simulink model "resultados_controle_FALA_tuned_PID"  (Simulink 8.7)
settings: Solver=ode45  StartTime=0.0  StopTime=260  FixedStep=0.01  MaxStep=0.1  RelTol=1e-3
InitFcn:
  | % load parameters of the default quadrotor
  | disp('Quadrotor parameters loaded by InitFcn')
  | load =250;
  | mdl_quadrotor
  | 
  | % --- Outer loop gains --------
  | %Versao 1
  | %P_X = 3.25; I_X = 0.45; D_X = 2;
  | %P_Y = 2.75; I_Y = 0.35; D_Y = 4.75;
  | %P_Z = 45;    I_Z = 3.5;   D_Z = 25;
  | 
  | %FALA TUNNED WITH LOAD
  | P_X = 9.2;      I_X = 0.16;     D_X  =  3.45;
  | P_Y = 8.9;      I_Y = 0.04;      D_Y  = 3.5;
  | P_Z = 53;       I_Z = 5.2;        D_Z = 26.7;
  | % --------------------------
undefined symbols (not defined in the file or in its folder): quad, sigbuilder_block
libraries: simulink_extras x5, dspsigops x4
settings Model: Creator=corkep  LastModifiedBy=kleber
settings DataIOCC: SignalLoggingSaveFormat=ModelDataLogs
settings OptimizationCC: ExpressionDepthLimit=2147483647
settings DebuggingCC: SolverPrmCheckMsg=warning  FcnCallInpInsideContextMsg=UseLocalSettings  StateNameClashWarn=warning
settings GRTTargetCC: CombineOutputUpdateFcns=off  GRTInterface=on
settings ConfigComp: CovSFcnEnable=off

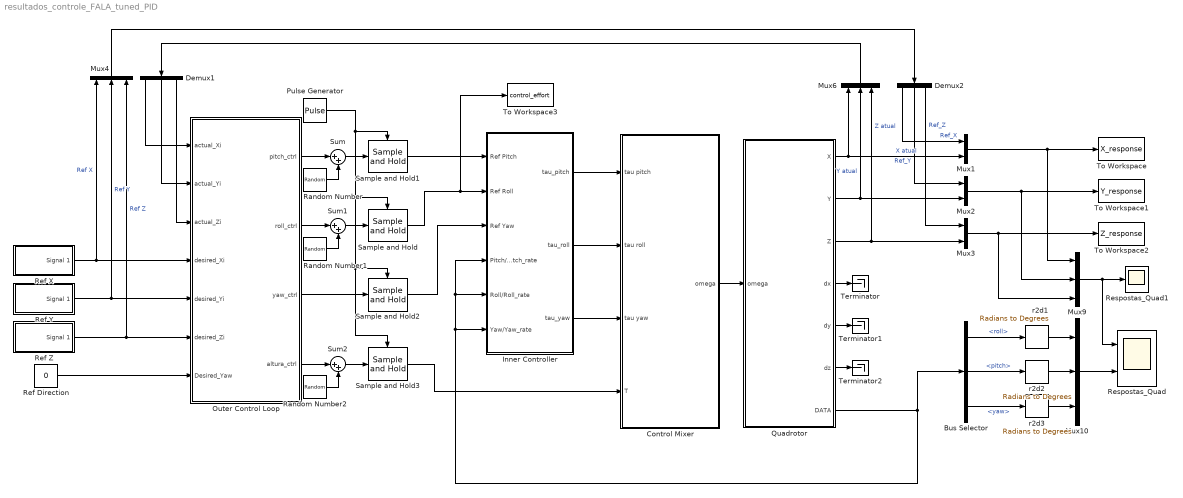
== system resultados_controle_FALA_tuned_PID ==
  Bus Selector : BusSelector  OutputSignals=roll,pitch,yaw
  Control Mixer : Subsystem  AncestorBlock=roblocks/Dynamics/Control Mixer 4
      mask help: Quadrotor control mixer
      mask Help:
      | Determine rotor speeds based on desired torques and thrust.
      | 
      | <b>Inputs::</b>
      | 
      | tau pitch (1x1)  desired pitching torque [Nm]
      | tau roll (1x1)   desired rolling torque [Nm]
      | tau yaw (1x1)    desired yawing torque [Nm]
      | T (1x1)          desired thrust [N]
      | 
      | <b>Outputs::</b>
      | 
      | w1 (1x1) angular velocity of rotor 1 [rad]
      | w2 (1x1) angular velocity of rotor 2 [rad]
      | w3 (1x1) angular velocity of rotor 3 [rad]
      | w4 (1x1) angular velocity of rotor 4 [rad]
      | 
      | <b>Notes::</b>
      | 
      | - Assumes the rotor labelling convention of RVC Fig 4.16.
      | - The quadrotor is underactuated and has only 4 inputs.
  Demux1 : Demux  Outputs=3
  Demux2 : Demux  Outputs=3
  Inner Controller : Subsystem
  Mux1 : Mux  Inputs=2
  Mux10 : Mux  Inputs=3
  Mux2 : Mux  Inputs=2
  Mux3 : Mux  Inputs=2
  Mux4 : Mux  Inputs=3
  Mux6 : Mux  RequirementInfo="{}  %GIDa_c1e701bd_0944_43f7_91ee_3360df493ed1"  Inputs=3
  Mux9 : Mux  Inputs=3
  Outer Control Loop : Subsystem
  Pulse Generator : DiscretePulseGenerator  PulseType=Time based  Period=0.1  PulseWidth=10
  Quadrotor : Subsystem  AncestorBlock=roblocks/Dynamics/Quadrotor  mask{quad=quad}
      mask prompts: quad "Quadrotor params"
      mask help: Quadrotor dynamics
      mask Help:
      | Integrate spatial velocity to update pose represented as a homogeneous
      | transformation.
      | 
      | <b>Parameters::</b>
      | 
      | q (struct)  A structure containing quadrotor dynamics
      | 
      | The elements of q are:
      | 
      |  J         Flyer rotational inertia matrix (3x3)
      |  h         Height of rotors above CoG (1x1)
      |  d         Length of flyer arms (1x1)
      |  nb        Number of blades per rotor (1x1)
      |  r         Rotor radius (1x1)
      |  c         Blade chord (1x1)
      |  e         Flapping hinge offset (1x1)
      |  Mb        Rotor blade mass (1x1)
      |  Mc        Estimated hub clamp mass (1x1)
      |  ec        Blade root clamp displacement (1x1)
      |  Ib        Rotor blade rotational inertia (1x1)
      |  Ic        Estimated root clamp inertia (1x1)
      |  mb        Static blade moment (1x1)
      |  Ir        Total rotor inertia (1x1)
      |  Ct        Non-dim. thrust coefficient (1x1)
      |  Cq        Non-dim. torque coefficient (1x1)
      |  sigma     Rotor solidity ratio (1x1)
      |  thetat    Blade tip angle (1x1)
      |  theta0    Blade root angle (1x1)
      |  theta1    Blade twist angle (1x1)
      |  theta75   3/4 blade angle (1x1)
      |  thetai    Blade ideal root approximation (1x1)
      |  a         Lift slope gradient (1x1)
      |  A         Rotor disc area (1x1)
      |  gamma     Lock number (1x1)
      | 
      | 
      | <b>Inputs::</b>
      | 
      | w1 (1x1) angular velocity of rotor 1 [rad]
      | w2 (1x1) angular velocity of rotor 2 [rad]
      | w3 (1x1) angular velocity of rotor 3 [rad]
      | w4 (1x1) angular velocity of rotor 4 [rad]
      | 
      | <b>Outputs::</b>
      | 
      | X (1x12) state vector (x, y, z, thr, thp, thy, xd, yd, zd, thrd, thpd, thyd)
      | 
      | (x,y,z) is the position in the world frame [m]
      | (thr, thp, thy) the roll/pitch/yaw orientation in the world frame [rad]
      | (xd,yd,zd) is the velocity in the body frame [m]
      | (thrd,thpd,thyd) is the roll/pitch/yaw rates in the body frame [rad/s]
      | 
      | <b>Notes::</b>
      | 
      | - See also mdl_quadrotor which defines parameters for the ANU X4 flyer.
  Random Number : RandomNumber  Variance=0.0001  SampleTime=0.01
  Random Number1 : RandomNumber  Variance=0.0001  SampleTime=0.01
  Random Number2 : RandomNumber  Variance=0.25  SampleTime=0.01
  Ref Direction : Constant  Value=0  SampleTime=0
  Ref X : Subsystem  Tag=STV Subsys  LoadFcn=sigbuilder_block('load');  StartFcn=sigbuilder_block('start');  StopFcn=sigbuilder_block('stop');  ClipboardFcn=sigbuilder_block('clipboard');  mask(Sigbuilder block){}
      mask help: Sigbuilder GUI
      mask init:
      | if ~strcmp(get_param(bdroot(gcbh),'SimulationStatus'),'stopped') tuvar = sigbuilder_block('maskInit'); end
      settings: CopyFcn=sigbuilder_block('copy');  DeleteFcn=sigbuilder_block('delete');  ModelCloseFcn=sigbuilder_block('modelClose');  PreSaveFcn=sigbuilder_block('preSave');  PauseFcn=sigbuilder_block('pause')  ContinueFcn=sigbuilder_block('continue')  NameChangeFcn=sigbuilder_block('namechange');  OpenFcn=sigbuilder_block('open',[156 64.5 984.75 417 ]);  CloseFcn=sigbuilder_block('close');
      mask Display: plot(0,0,100,100,[10,10,40,40,10],[80,20,20,80,80],[40,10],[50,50], [40,27,10],[65,72,56],[40,25,25,10],[28,28,43,43]);
  Ref Y : Subsystem  Tag=STV Subsys  LoadFcn=sigbuilder_block('load');  StartFcn=sigbuilder_block('start');  StopFcn=sigbuilder_block('stop');  ClipboardFcn=sigbuilder_block('clipboard');  mask(Sigbuilder block){}
      mask help: Sigbuilder GUI
      mask init:
      | if ~strcmp(get_param(bdroot(gcbh),'SimulationStatus'),'stopped') tuvar = sigbuilder_block('maskInit'); end
      settings: CopyFcn=sigbuilder_block('copy');  DeleteFcn=sigbuilder_block('delete');  ModelCloseFcn=sigbuilder_block('modelClose');  PreSaveFcn=sigbuilder_block('preSave');  PauseFcn=sigbuilder_block('pause')  ContinueFcn=sigbuilder_block('continue')  NameChangeFcn=sigbuilder_block('namechange');  OpenFcn=sigbuilder_block('open',[166.5 -89.25 984.75 454.5 ]);  CloseFcn=sigbuilder_block('close');
      mask Display: plot(0,0,100,100,[10,10,40,40,10],[80,20,20,80,80],[40,10],[50,50], [40,27,10],[65,72,56],[40,25,25,10],[28,28,43,43]);
  Ref Z : Subsystem  Tag=STV Subsys  LoadFcn=sigbuilder_block('load');  StartFcn=sigbuilder_block('start');  StopFcn=sigbuilder_block('stop');  ClipboardFcn=sigbuilder_block('clipboard');  mask(Sigbuilder block){}
      mask help: Sigbuilder GUI
      mask init:
      | if ~strcmp(get_param(bdroot(gcbh),'SimulationStatus'),'stopped') tuvar = sigbuilder_block('maskInit'); end
      settings: CopyFcn=sigbuilder_block('copy');  DeleteFcn=sigbuilder_block('delete');  ModelCloseFcn=sigbuilder_block('modelClose');  PreSaveFcn=sigbuilder_block('preSave');  PauseFcn=sigbuilder_block('pause')  ContinueFcn=sigbuilder_block('continue')  NameChangeFcn=sigbuilder_block('namechange');  OpenFcn=sigbuilder_block('open',[39.75 32.25 984.75 237.75 ]);  CloseFcn=sigbuilder_block('close');
      mask Display: plot(0,0,100,100,[10,10,40,40,10],[80,20,20,80,80],[40,10],[50,50], [40,27,10],[65,72,56],[40,25,25,10],[28,28,43,43]);
  Respostas_Quad : Scope  NumInputPorts=2
  Respostas_Quad1 : Scope
  Sample and Hold{,1..3} (4 alike) : dspsigops/Sample and Hold  trig=Rising edge  initCond=0  latchinput=off
  Sum : Sum  Inputs=|++
  Sum1 : Sum  Inputs=|++
  Sum2 : Sum  Inputs=|++
  Terminator : Terminator
  Terminator1 : Terminator
  Terminator2 : Terminator
  To Workspace : ToWorkspace  VariableName=X_response  SampleTime=-1
      settings: Save2DSignal=2-D array (concatenate along first dimension)
  To Workspace1 : ToWorkspace  VariableName=Y_response  SampleTime=-1
      settings: Save2DSignal=2-D array (concatenate along first dimension)
  To Workspace2 : ToWorkspace  VariableName=Z_response  SampleTime=-1
      settings: Save2DSignal=2-D array (concatenate along first dimension)
  To Workspace3 : ToWorkspace  VariableName=control_effort  SampleTime=-1
      settings: Save2DSignal=2-D array (concatenate along first dimension)
  r2d1 : simulink_extras/Transformations/Radians to Degrees
  r2d2 : simulink_extras/Transformations/Radians to Degrees
  r2d3 : simulink_extras/Transformations/Radians to Degrees
  wires:
  Quadrotor/7(DATA) -> Bus Selector/1, Inner Controller/6(Yaw/Yaw_rate), Inner Controller/5(Roll/Roll_rate), Inner Controller/4(Pitch/Pitch_rate)
  Sample and Hold3/1 -> Control Mixer/4(T)
  Control Mixer/1(omega) -> Quadrotor/1(omega)
  Ref Z/1(Signal 1) -> Outer Control Loop/6(desired_Zi), Mux4/3  "Ref Z"
  Ref Direction/1 -> Outer Control Loop/7(Desired_Yaw)
  Sample and Hold2/1 -> Inner Controller/3(Ref Yaw)
  Ref Y/1(Signal 1) -> Mux4/2, Outer Control Loop/5(desired_Yi)  "Ref Y"
  Mux2/1 -> To Workspace1/1, Mux9/2
  Demux2/1 -> Mux1/1  "Ref_X"
  Demux2/2 -> Mux2/1  "Ref_Y"
  Demux2/3 -> Mux3/1  "Ref_Z"
  Mux4/1 -> Demux2/1
  Pulse Generator/1 -> Sample and Hold1/Trigger, Sample and Hold/Trigger, Sample and Hold2/Trigger, Sample and Hold3/Trigger
  Mux9/1 -> Respostas_Quad1/1, Respostas_Quad/1
  Mux10/1 -> Respostas_Quad/2
  Bus Selector/2 -> r2d2/1  "<pitch>"
  Bus Selector/1 -> r2d1/1  "<roll>"
  Quadrotor/1(X) -> Mux1/2, Mux6/1  "X atual"
  Quadrotor/3(Z) -> Mux3/2, Mux6/3  "Z atual"
  Bus Selector/3 -> r2d3/1  "<yaw>"
  Quadrotor/2(Y) -> Mux2/2, Mux6/2  "Y atual"
  Sample and Hold1/1 -> Inner Controller/1(Ref Pitch)
  Quadrotor/4(dx) -> Terminator/1
  Quadrotor/5(dy) -> Terminator1/1
  Quadrotor/6(dz) -> Terminator2/1
  Mux6/1 -> Demux1/1
  Demux1/1 -> Outer Control Loop/1(actual_Xi)
  Demux1/2 -> Outer Control Loop/2(actual_Yi)
  Demux1/3 -> Outer Control Loop/3(actual_Zi)
  Mux3/1 -> To Workspace2/1, Mux9/3
  Inner Controller/2(tau_roll) -> Control Mixer/2(tau roll)
  Inner Controller/3(tau_yaw) -> Control Mixer/3(tau yaw)
  r2d1/1 -> Mux10/1
  r2d2/1 -> Mux10/2
  r2d3/1 -> Mux10/3
  Inner Controller/1(tau_pitch) -> Control Mixer/1(tau pitch)
  Ref X/1(Signal 1) -> Outer Control Loop/4(desired_Xi), Mux4/1  "Ref X"
  Random Number2/1 -> Sum2/2
  Random Number1/1 -> Sum1/2
  Random Number/1 -> Sum/2
  Outer Control Loop/1(pitch_ctrl) -> Sum/1
  Sum/1 -> Sample and Hold1/1
  Outer Control Loop/2(roll_ctrl) -> Sum1/1
  Sum1/1 -> Sample and Hold/1
  Sample and Hold/1 -> To Workspace3/1, Inner Controller/2(Ref Roll)
  Sum2/1 -> Sample and Hold3/1
  Outer Control Loop/4(altura_ctrl) -> Sum2/1
  Outer Control Loop/3(yaw_ctrl) -> Sample and Hold2/1
  Mux1/1 -> To Workspace/1, Mux9/1

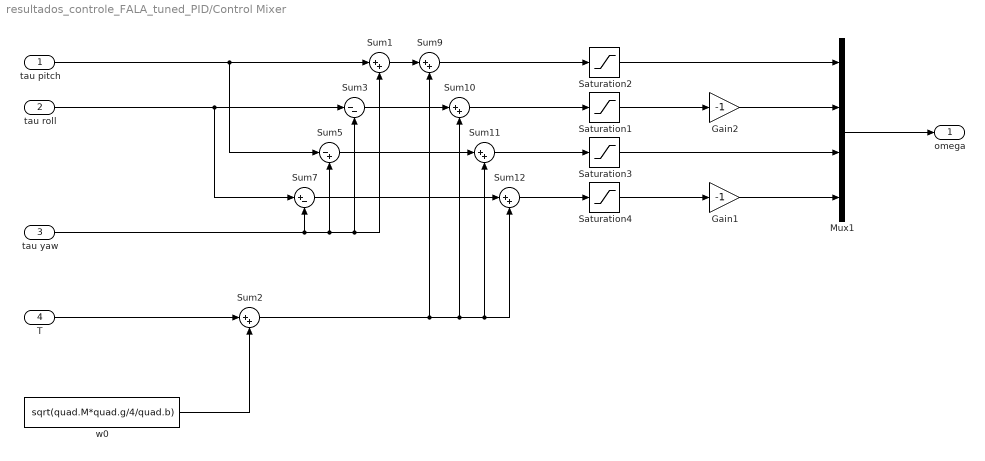
== system resultados_controle_FALA_tuned_PID/Control Mixer ==
  tau pitch : Inport
  tau roll : Inport  Port=2
  tau yaw : Inport  Port=3
  T : Inport  Port=4
  Gain1 : Gain  Gain=-1
  Gain2 : Gain  Gain=-1
  Mux1 : Mux
  Saturation{1..4} (4 alike) : Saturate  UpperLimit=1000  LowerLimit=700
  Sum{1..2,9..12} (6 alike) : Sum  Inputs=|++  SaturateOnIntegerOverflow=on  InputSameDT=on  OutDataTypeStr=Inherit: Same as first input
  Sum3 : Sum  Inputs=|--  SaturateOnIntegerOverflow=on  InputSameDT=on  OutDataTypeStr=Inherit: Same as first input
  Sum5 : Sum  Inputs=|-+  SaturateOnIntegerOverflow=on  InputSameDT=on  OutDataTypeStr=Inherit: Same as first input
  Sum7 : Sum  Inputs=|+-  SaturateOnIntegerOverflow=on  InputSameDT=on  OutDataTypeStr=Inherit: Same as first input
  w0 : Constant  Value=sqrt(quad.M*quad.g/4/quad.b)  SampleTime=0
  omega : Outport
  wires:
  Mux1/1 -> omega/1
  Gain2/1 -> Mux1/2
  tau yaw/1 -> Sum7/2, Sum5/2, Sum3/2, Sum1/2
  Saturation2/1 -> Mux1/1
  Saturation1/1 -> Gain2/1
  Saturation3/1 -> Mux1/3
  Saturation4/1 -> Gain1/1
  tau pitch/1 -> Sum5/1, Sum1/1
  Sum1/1 -> Sum9/1
  Sum3/1 -> Sum10/1
  Sum5/1 -> Sum11/1
  Sum7/1 -> Sum12/1
  Sum9/1 -> Saturation2/1
  Sum10/1 -> Saturation1/1
  Sum11/1 -> Saturation3/1
  Sum12/1 -> Saturation4/1
  tau roll/1 -> Sum7/1, Sum3/1
  Gain1/1 -> Mux1/4
  Sum2/1 -> Sum9/2, Sum11/2, Sum12/2, Sum10/2
  T/1 -> Sum2/1
  w0/1 -> Sum2/2

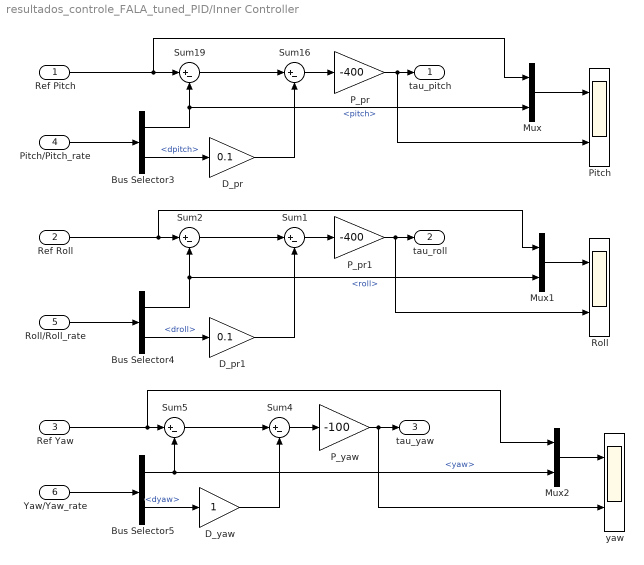
== system resultados_controle_FALA_tuned_PID/Inner Controller ==
  Ref Pitch : Inport
  Ref Roll : Inport  Port=2
  Ref Yaw : Inport  Port=3
  Pitch/Pitch_rate : Inport  Port=4
  Roll/Roll_rate : Inport  Port=5
  Yaw/Yaw_rate : Inport  Port=6
  Bus Selector3 : BusSelector  OutputSignals=pitch,dpitch
  Bus Selector4 : BusSelector  OutputSignals=roll,droll
  Bus Selector5 : BusSelector  OutputSignals=yaw,dyaw
  D_pr : Gain  Gain=0.1
  D_pr1 : Gain  Gain=0.1
  D_yaw : Gain
  Mux : Mux  Inputs=2
  Mux1 : Mux  Inputs=2
  Mux2 : Mux  Inputs=2
  P_pr : Gain  Gain=-400
  P_pr1 : Gain  Gain=-400
  P_yaw : Gain  Gain=-100
  Pitch : Scope  NumInputPorts=2
  Roll : Scope  NumInputPorts=2
  Sum{1..2,4..5,16,19} (6 alike) : Sum  Inputs=|+-
  yaw : Scope  NumInputPorts=2
  tau_pitch : Outport
  tau_roll : Outport  Port=2
  tau_yaw : Outport  Port=3
  wires:
  Sum19/1 -> Sum16/1
  Sum16/1 -> P_pr/1
  P_pr/1 -> Pitch/2, tau_pitch/1
  D_pr/1 -> Sum16/2
  Bus Selector3/2 -> D_pr/1  "<dpitch>"
  Bus Selector3/1 -> Sum19/2, Mux/2  "<pitch>"
  Sum2/1 -> Sum1/1
  Sum1/1 -> P_pr1/1
  P_pr1/1 -> Roll/2, tau_roll/1
  D_pr1/1 -> Sum1/2
  Bus Selector4/2 -> D_pr1/1  "<droll>"
  Ref Pitch/1 -> Mux/1, Sum19/1
  Pitch/Pitch_rate/1 -> Bus Selector3/1
  Roll/Roll_rate/1 -> Bus Selector4/1
  Bus Selector4/1 -> Mux1/2, Sum2/2  "<roll>"
  Ref Roll/1 -> Mux1/1, Sum2/1
  Bus Selector5/1 -> Sum5/2, Mux2/2  "<yaw>"
  Sum4/1 -> P_yaw/1
  Bus Selector5/2 -> D_yaw/1  "<dyaw>"
  D_yaw/1 -> Sum4/2
  Sum5/1 -> Sum4/1
  P_yaw/1 -> yaw/2, tau_yaw/1
  Yaw/Yaw_rate/1 -> Bus Selector5/1
  Ref Yaw/1 -> Mux2/1, Sum5/1
  Mux/1 -> Pitch/1
  Mux1/1 -> Roll/1
  Mux2/1 -> yaw/1

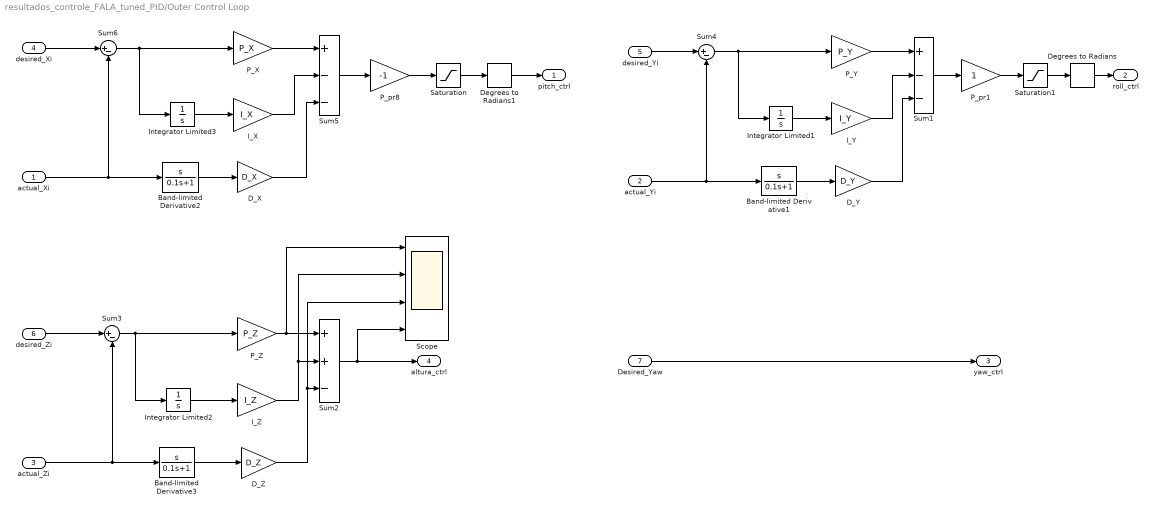
== system resultados_controle_FALA_tuned_PID/Outer Control Loop ==
  actual_Xi : Inport
  actual_Yi : Inport  Port=2
  actual_Zi : Inport  Port=3
  desired_Xi : Inport  Port=4
  desired_Yi : Inport  Port=5
  desired_Zi : Inport  Port=6
  Desired_Yaw : Inport  Port=7
  Band-limited Deriv ative1 : TransferFcn  Numerator=[1 0]  Denominator=[0.1 1]
  Band-limited Derivative2 : TransferFcn  Numerator=[1 0]  Denominator=[0.1 1]
  Band-limited Derivative3 : TransferFcn  Numerator=[1 0]  Denominator=[0.1 1]
  D_X : Gain  Gain=D_X
  D_Y : Gain  Gain=D_Y
  D_Z : Gain  Gain=D_Z
  Degrees to Radians : simulink_extras/Transformations/Degrees to Radians
  Degrees to Radians1 : simulink_extras/Transformations/Degrees to Radians
  I_X : Gain  Gain=I_X
  I_Y : Gain  Gain=I_Y
  I_Z : Gain  Gain=I_Z
  Integrator Limited1 : Integrator  LimitOutput=on  UpperSaturationLimit=0.5  LowerSaturationLimit=-0.5
  Integrator Limited2 : Integrator  LimitOutput=on  UpperSaturationLimit=10  LowerSaturationLimit=0
  Integrator Limited3 : Integrator  LimitOutput=on  UpperSaturationLimit=0.5  LowerSaturationLimit=-0.5
  P_X : Gain  Gain=P_X
  P_Y : Gain  Gain=P_Y
  P_Z : Gain  Gain=P_Z
  P_pr1 : Gain
  P_pr8 : Gain  Gain=-1
  Saturation : Saturate  UpperLimit=2  LowerLimit=-2
  Saturation1 : Saturate  UpperLimit=2  LowerLimit=-2
  Scope : Scope  NumInputPorts=4
  Sum1 : Sum  Inputs=+--
  Sum2 : Sum  Inputs=++-
  Sum3 : Sum  Inputs=|+-
  Sum4 : Sum  Inputs=|+-
  Sum5 : Sum  Inputs=+--
  Sum6 : Sum  Inputs=|+-
  pitch_ctrl : Outport
  roll_ctrl : Outport  Port=2
  yaw_ctrl : Outport  Port=3
  altura_ctrl : Outport  Port=4
  wires:
  Sum3/1 -> Integrator Limited2/1, P_Z/1
  Integrator Limited2/1 -> I_Z/1
  P_Z/1 -> Sum2/1, Scope/1
  D_Z/1 -> Scope/3, Sum2/3
  actual_Zi/1 -> Sum3/2, Band-limited Derivative3/1
  Band-limited Derivative3/1 -> D_Z/1
  desired_Zi/1 -> Sum3/1
  Desired_Yaw/1 -> yaw_ctrl/1
  Sum6/1 -> Integrator Limited3/1, P_X/1
  Integrator Limited3/1 -> I_X/1
  P_X/1 -> Sum5/1
  D_X/1 -> Sum5/3
  actual_Xi/1 -> Band-limited Derivative2/1, Sum6/2
  Band-limited Derivative2/1 -> D_X/1
  desired_Xi/1 -> Sum6/1
  I_X/1 -> Sum5/2
  Sum4/1 -> Integrator Limited1/1, P_Y/1
  Integrator Limited1/1 -> I_Y/1
  P_Y/1 -> Sum1/1
  D_Y/1 -> Sum1/3
  actual_Yi/1 -> Sum4/2, Band-limited Deriv ative1/1
  Band-limited Deriv ative1/1 -> D_Y/1
  desired_Yi/1 -> Sum4/1
  I_Y/1 -> Sum1/2
  Degrees to Radians/1 -> roll_ctrl/1
  Degrees to Radians1/1 -> pitch_ctrl/1
  Sum1/1 -> P_pr1/1
  I_Z/1 -> Sum2/2, Scope/2
  Sum5/1 -> P_pr8/1
  Sum2/1 -> Scope/4, altura_ctrl/1
  P_pr8/1 -> Saturation/1
  Saturation/1 -> Degrees to Radians1/1
  P_pr1/1 -> Saturation1/1
  Saturation1/1 -> Degrees to Radians/1

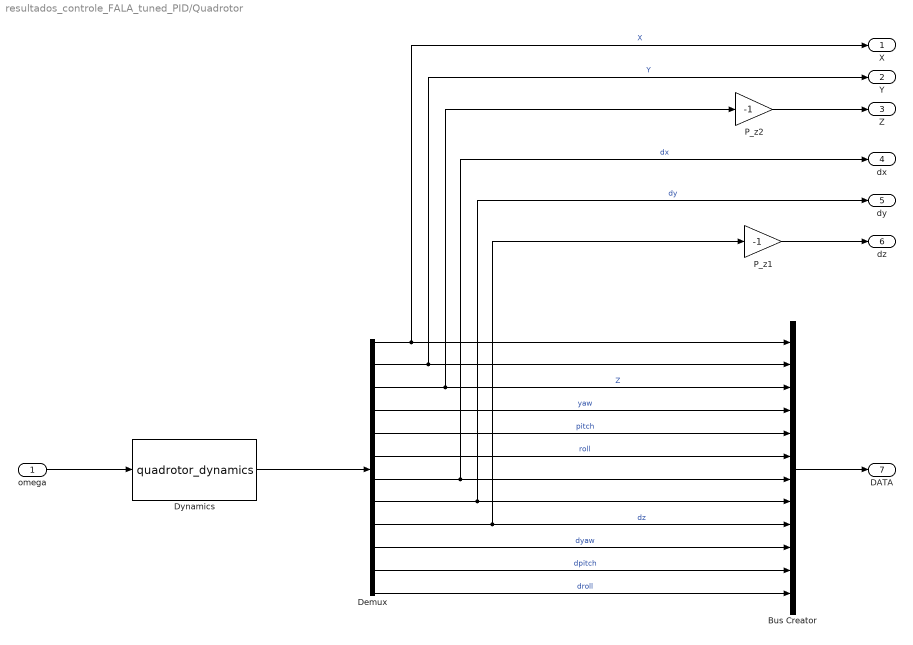
== system resultados_controle_FALA_tuned_PID/Quadrotor ==
  omega : Inport
  Bus Creator : BusCreator  Inputs='X','Y','Z','yaw','pitch','roll','dx','dy','dz','dyaw','dpitch','droll'
  Demux : Demux  Outputs=12
  Dynamics : S-Function  FunctionName=quadrotor_dynamics  Parameters=quad  SFunctionDeploymentMode=off  EnableBusSupport=off
  P_z1 : Gain  Gain=-1
  P_z2 : Gain  Gain=-1
  X : Outport
  Y : Outport  Port=2
  Z : Outport  Port=3
  dx : Outport  Port=4
  dy : Outport  Port=5
  dz : Outport  Port=6
  DATA : Outport  Port=7
  wires:
  Demux/1 -> X/1, Bus Creator/1  "X"
  Demux/3 -> Bus Creator/3, P_z2/1  "Z"
  Demux/4 -> Bus Creator/4  "yaw"
  Demux/5 -> Bus Creator/5  "pitch"
  omega/1 -> Dynamics/1
  Demux/7 -> dx/1, Bus Creator/7  "dx"
  Demux/9 -> P_z1/1, Bus Creator/9  "dz"
  Demux/2 -> Y/1, Bus Creator/2  "Y"
  Demux/6 -> Bus Creator/6  "roll"
  Demux/8 -> dy/1, Bus Creator/8  "dy"
  Bus Creator/1 -> DATA/1
  Dynamics/1 -> Demux/1
  Demux/10 -> Bus Creator/10  "dyaw"
  Demux/11 -> Bus Creator/11  "dpitch"
  Demux/12 -> Bus Creator/12  "droll"
  P_z2/1 -> Z/1
  P_z1/1 -> dz/1

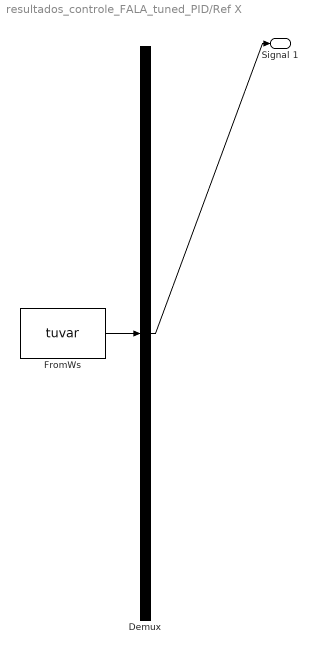
== system resultados_controle_FALA_tuned_PID/Ref X ==
  Demux : Demux  Tag=STV Demux  Outputs=1
  FromWs : FromWorkspace  Tag=STV FromWs  VariableName=tuvar  SampleTime=0  SigBuilderData=DataTag0  VnvData=DataTag1
      SigBuilderData=|
      | common.afterFinalStr = 'Extrapolate'
      | common.sampleTime = 0
      | dataSet.timeRange = [0 300]
      | dataSet.name = 'Group 1'
      | sbobj.Name = 'Signal Builder'
      | sbobj.Groups.Name = 'Group 1'
      | sbobj.Groups.Signals.Name = 'Signal 1'
      | sbobj.Groups.Signals.XData = [0 10 20 120 125 300]
      | sbobj.Groups.Signals.YData = [0 0 1 1 1.5 1.5]
      | sbobj.Groups.TimeRange = [0 300]
  Signal 1 : Outport  Tag=STV Outport
  wires:
  FromWs/1 -> Demux/1
  Demux/1 -> Signal 1/1

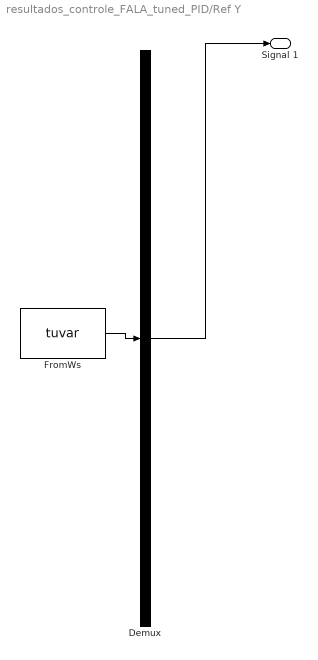
== system resultados_controle_FALA_tuned_PID/Ref Y ==
  Demux : Demux  Tag=STV Demux  Outputs=1
  FromWs : FromWorkspace  Tag=STV FromWs  VariableName=tuvar  SampleTime=0  SigBuilderData=DataTag2  VnvData=DataTag3
      SigBuilderData=|
      | common.afterFinalStr = 'Extrapolate'
      | common.sampleTime = 0
      | dataSet.timeRange = [0 300]
      | dataSet.name = 'Group 1'
      | sbobj.Name = 'Signal Builder'
      | sbobj.Groups.Name = 'Group 1'
      | sbobj.Groups.Signals.Name = 'Signal 1'
      | sbobj.Groups.Signals.XData = [0 10 20 50 70 120 140 190 210 300]
      | sbobj.Groups.Signals.YData = [0 0 0.5 0.5 2.5 2.5 0.5 0.5 2.5 2.5]
      | sbobj.Groups.TimeRange = [0 300]
  Signal 1 : Outport  Tag=STV Outport
  wires:
  FromWs/1 -> Demux/1
  Demux/1 -> Signal 1/1

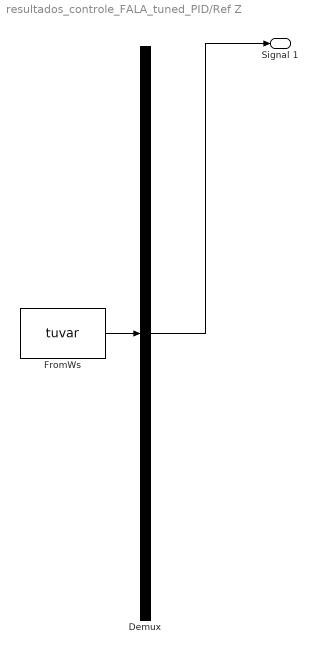
== system resultados_controle_FALA_tuned_PID/Ref Z ==
  Demux : Demux  Tag=STV Demux  Outputs=1
  FromWs : FromWorkspace  Tag=STV FromWs  VariableName=tuvar  SampleTime=0  SigBuilderData=DataTag4  VnvData=DataTag5
      SigBuilderData=|
      | common.afterFinalStr = 'Extrapolate'
      | common.sampleTime = 0
      | dataSet.timeRange = [0 300]
      | dataSet.name = 'Group 1'
      | sbobj.Name = 'Signal Builder'
      | sbobj.Groups.Name = 'Group 1'
      | sbobj.Groups.Signals.Name = 'Signal 1'
      | sbobj.Groups.Signals.XData = [0 5 25 35 40 50 85 95 100 110 155 165 170 180 225 235 240 250 300]
      | sbobj.Groups.Signals.YData = [0.15 0.5 0.5 0.15 0.15 0.5 0.5 0.15 0.15 0.5 0.5 0.15 0.15 0.5 0.5 0.15 0.15 0.5 0.5]
      | sbobj.Groups.TimeRange = [0 300]
  Signal 1 : Outport  Tag=STV Outport
  wires:
  FromWs/1 -> Demux/1
  Demux/1 -> Signal 1/1
